simulink model "model"  (R2023a)
settings: Solver=ode4  StartTime=0.0  StopTime=5  FixedStep=0.01  RelTol=1e-3
undefined symbols (not defined in the file or in its folder): b_c, k_c, t_fc
settings Model: Creator=ADMIN  LastModifiedBy=ADMIN

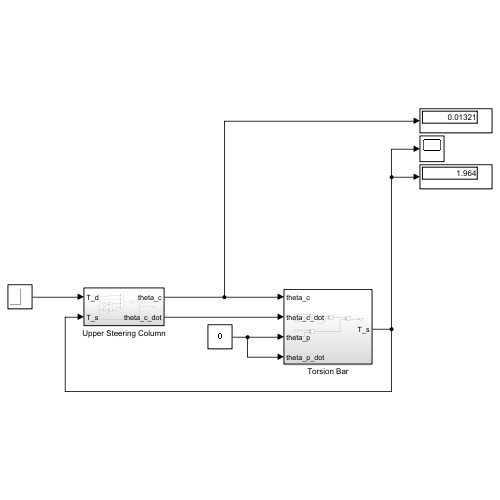
[thumbnail: Simulink's stored preview of the top-level diagram]
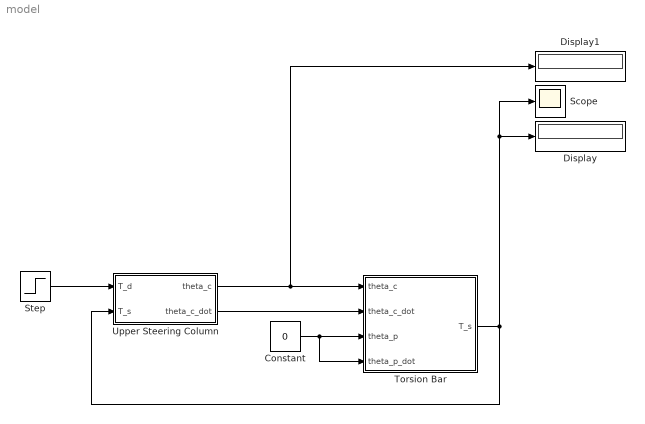
== system model ==
  Constant : Constant  Value=0
  Display : Display
  Display1 : Display
  Scope : Scope
  Step : Step  After=2  SampleTime=0
  Torsion Bar : Subsystem
  Upper Steering Column : Subsystem
  wires:
  Upper Steering Column/1(theta_c) -> Display1/1, Torsion Bar/1(theta_c)
  Upper Steering Column/2(theta_c_dot) -> Torsion Bar/2(theta_c_dot)
  Constant/1 -> Torsion Bar/4(theta_p_dot), Torsion Bar/3(theta_p)
  Step/1 -> Upper Steering Column/1(T_d)
  Torsion Bar/1(T_s) -> Scope/1, Display/1, Upper Steering Column/2(T_s)

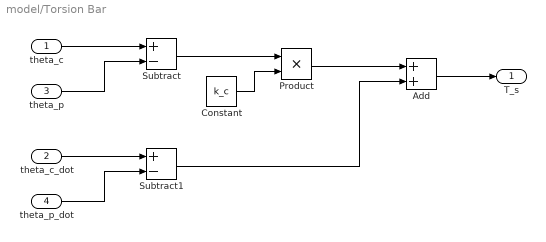
== system model/Torsion Bar ==
  theta_c : Inport
  theta_c_dot : Inport  Port=2
  theta_p : Inport  Port=3
  theta_p_dot : Inport  Port=4
  Add : Sum
  Constant : Constant  Value=k_c
  Product : Product
  Subtract : Sum  Inputs=+-
  Subtract1 : Sum  Inputs=+-
  T_s : Outport
  wires:
  theta_c/1 -> Subtract/1
  theta_p/1 -> Subtract/2
  Subtract/1 -> Product/1
  Constant/1 -> Product/2
  Product/1 -> Add/1
  Add/1 -> T_s/1
  theta_c_dot/1 -> Subtract1/1
  theta_p_dot/1 -> Subtract1/2
  Subtract1/1 -> Add/2

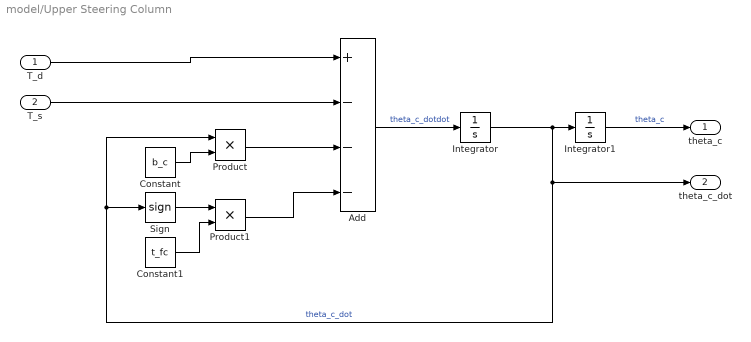
== system model/Upper Steering Column ==
  T_d : Inport
  T_s : Inport  Port=2
  Add : Sum  Inputs=+---
  Constant : Constant  Value=b_c
  Constant1 : Constant  Value=t_fc
  Integrator : Integrator
  Integrator1 : Integrator
  Product : Product
  Product1 : Product
  Sign : Signum
  theta_c : Outport
  theta_c_dot : Outport  Port=2
  wires:
  T_d/1 -> Add/1
  T_s/1 -> Add/2
  Constant/1 -> Product/2
  Product/1 -> Add/3
  Add/1 -> Integrator/1  "theta_c_dotdot"
  Integrator/1 -> Integrator1/1, Product/1, Sign/1, theta_c_dot/1  "theta_c_dot"
  Integrator1/1 -> theta_c/1  "theta_c"
  Constant1/1 -> Product1/2
  Product1/1 -> Add/4
  Sign/1 -> Product1/1
